simulink model "sysgenQAMExt"  (Simulink 7.7)
settings: Solver=ode45  StartTime=0.0  StopTime=3000  RelTol=1e-3
PreLoadFcn:
  | xlrequire('PreLoadFcn')
values from neighbouring files (symbols this model uses):
  hh = hh1/max(hh1)    [sysgenCostasLoop_PreLoadFcn.m]
  j = find(xLabel==')')    [sdspfscope2_r13.m]
  k = (k-1)*3+2    [sdspfscope2_r13.m]
  mu = xfix({xlSigned, 18, 15, xlRound, xlSaturate}, mu)    [lmsErr.m]
undefined symbols (not defined in the file or in its folder): chan, k_i0, k_p0, xlipgetpartsetting, xlsfunxy
libraries: xbsIndex_r4 x477, simulink x2, dspsigops x2, dspmlti4 x2, commchan3 x1, xbsCopyrightNotice_r4 x1, dspobslib x1
(part 2 of 5)

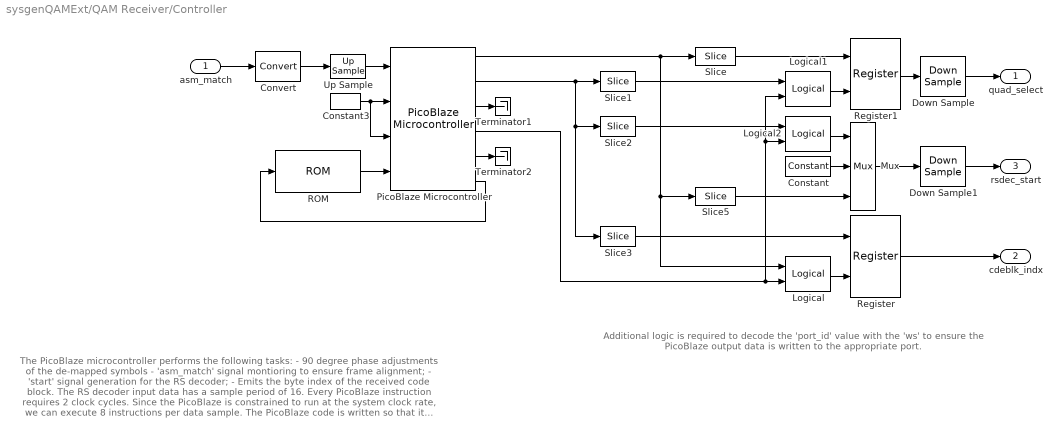
== system sysgenQAMExt/QAM Receiver/Controller ==
  note: The PicoBlaze microcontroller performs the following tasks:
      |
      | - 90 degree phase adjustments of the de-mapped symbols
      | - 'asm_match' signal montioring to ensure frame alignment;
      | - 'start' signal generation for the RS decoder;
      | - Emits the byte index of the received code block.
      |
      | The RS decoder input data has a sample period of 16.
      | Every PicoBlaze instruction requires 2 clock cycles.  Since
      | the PicoBlaze is constrained to run at the system clock rate,
      | we can execute 8 instructions per data sample.  The
      | PicoBlaze code is  written so that it remains synchronized
      | with the data, i.e. there are exactly eight instructions between
      | input samples.
      |
      | Please refer to the PicoBlaze code, sysgenQAMExt.psm for
      | more information.
  note: Additional logic is required to decode the
      | 'port_id' value with the 'ws' to ensure
      | the PicoBlaze output data is written
      | to the appropriate port.
  asm_match : Inport
  Constant : xbsIndex_r4/Constant  const=0  gui_display_data_type=Fixed-point  arith_type=Boolean  n_bits=1  bin_pt=0  preci_type=Single  exp_width=8  frac_width=24  explicit_period=off  period=1  equ=P=C  opselect=C  inp2=PCIN>>17  opr=+  inp1=P  carry=CIN  dbl_ovrd=off  block_type=constant
      settings: block_version=VER_STRING_GOES_HERE
  Constant3 : xbsIndex_r4/Constant  const=0  gui_display_data_type=Fixed-point  arith_type=Boolean  n_bits=1  bin_pt=0  preci_type=Single  exp_width=8  frac_width=24  explicit_period=on  period=1  equ=P=C  opselect=C  inp2=PCIN>>17  opr=+  inp1=P  carry=CIN  dbl_ovrd=off  block_type=constant
      settings: block_version=VER_STRING_GOES_HERE
  Convert : xbsIndex_r4/Convert  gui_display_data_type=Fixed-point  arith_type=Unsigned  n_bits=8  bin_pt=0  float_type=Single  exp_bits=8  fraction_bits=24  quantization=Truncate  overflow=Wrap  en=off  latency=0  dbl_ovrd=off  pipeline=off  block_type=convert
      settings: infoedit=The input is presented at the output after quantization and overflow effects.<P><P>Hardware notes: Additional hardware is used when rounding or saturation is selected and output width is less than the input width.  xl_area=[0, 0, 0, 0, 0, 0, 0]  block_version=VER_STRING_GOES_HERE
  Down Sample : xbsIndex_r4/Down Sample  sample_ratio=4  sample_phase="Last Value of Frame  (most efficient)"  en=off  latency=1  dbl_ovrd=off  block_type=dsamp
      settings: xl_area=[0, 0, 0, 0, 0, 0, 0]  block_version=VER_STRING_GOES_HERE
  Down Sample1 : xbsIndex_r4/Down Sample  sample_ratio=16  sample_phase="Last Value of Frame  (most efficient)"  en=off  latency=1  dbl_ovrd=off  block_type=dsamp
      settings: xl_area=[0, 0, 0, 0, 0, 0, 0]  block_version=VER_STRING_GOES_HERE
  Logical : xbsIndex_r4/Logical  logical_function=AND  inputs=2  en=off  latency=0  precision=Full  arith_type=Unsigned  n_bits=8  bin_pt=2  align_bp=on  dbl_ovrd=off  block_type=logical
      settings: xl_area=[0, 0, 0, 0, 0, 0, 0]  block_version=VER_STRING_GOES_HERE
  Logical1 : xbsIndex_r4/Logical  logical_function=AND  inputs=2  en=off  latency=0  precision=Full  arith_type=Unsigned  n_bits=8  bin_pt=2  align_bp=on  dbl_ovrd=off  block_type=logical
      settings: xl_area=[0, 0, 0, 0, 0, 0, 0]  block_version=VER_STRING_GOES_HERE
  Logical2 : xbsIndex_r4/Logical  logical_function=AND  inputs=2  en=off  latency=0  precision=Full  arith_type=Unsigned  n_bits=8  bin_pt=2  align_bp=on  dbl_ovrd=off  block_type=logical
      settings: xl_area=[0, 0, 0, 0, 0, 0, 0]  block_version=VER_STRING_GOES_HERE
  Mux : xbsIndex_r4/Mux  inputs=2  en=off  latency=0  precision=Full  arith_type="Signed  (2's comp)"  n_bits=8  bin_pt=2  quantization=Truncate  overflow=Wrap  dbl_ovrd=off  block_type=mux
      settings: xl_area=[0, 0, 0, 0, 0, 0, 0]  block_version=VER_STRING_GOES_HERE
  PicoBlaze Microcontroller : xbsIndex_r4/PicoBlaze Microcontroller  version=PicoBlaze 3  display_mi=off  xl_view_as=Decimal  block_type=pb
      settings: xl_area=[0, 0, 0, 0, 0, 0, 0]  block_version=VER_STRING_GOES_HERE
  ROM : xbsIndex_r4/ROM  depth=2^10  initVector=sysgenQAMExt_PBInstructs  distributed_mem=Block RAM  rst=off  init_reg=0  en=off  latency=1  gui_display_data_type=Fixed-point  arith_type=Unsigned  n_bits=18  bin_pt=0  preci_type=Single  exp_width=8  frac_width=24  dbl_ovrd=off  optimize=Area  use_rpm=off  block_type=sprom
      settings: xl_area=[0, 0, 0, 0, 0, 0, 0]  block_version=VER_STRING_GOES_HERE
  Register : xbsIndex_r4/Register  init=0  rst=off  en=on  dbl_ovrd=off  block_type=register
      settings: xl_area=[0, 0, 0, 0, 0, 0, 0]  block_version=VER_STRING_GOES_HERE
  Register1 : xbsIndex_r4/Register  init=0  rst=off  en=on  dbl_ovrd=off  block_type=register
      settings: xl_area=[0, 0, 0, 0, 0, 0, 0]  block_version=VER_STRING_GOES_HERE
  Slice : xbsIndex_r4/Slice  nbits=2  boolean_output=off  mode=Lower Bit Location + Width  bit1=0  base1=MSB of Input  bit0=0  base0=LSB of Input  dbl_ovrd=off  block_type=slice
      settings: infoedit="Extracts a given range of bits from each input sample and presents it at the output.  The output type is ordinarily unsigned with binary point at zero, but can be Boolean when the slice is one bit wide.<P><P>Hardware notes: In hardware this block costs nothing."  block_version=VER_STRING_GOES_HERE
  Slice1 : xbsIndex_r4/Slice  nbits=1  boolean_output=on  mode=Lower Bit Location + Width  bit1=0  base1=MSB of Input  bit0=0  base0=LSB of Input  dbl_ovrd=off  block_type=slice
      settings: infoedit="Extracts a given range of bits from each input sample and presents it at the output.  The output type is ordinarily unsigned with binary point at zero, but can be Boolean when the slice is one bit wide.<P><P>Hardware notes: In hardware this block costs nothing."  block_version=VER_STRING_GOES_HERE
  Slice2 : xbsIndex_r4/Slice  nbits=1  boolean_output=on  mode=Lower Bit Location + Width  bit1=0  base1=MSB of Input  bit0=1  base0=LSB of Input  dbl_ovrd=off  block_type=slice
      settings: infoedit="Extracts a given range of bits from each input sample and presents it at the output.  The output type is ordinarily unsigned with binary point at zero, but can be Boolean when the slice is one bit wide.<P><P>Hardware notes: In hardware this block costs nothing."  block_version=VER_STRING_GOES_HERE
  Slice3 : xbsIndex_r4/Slice  nbits=1  boolean_output=on  mode=Lower Bit Location + Width  bit1=0  base1=MSB of Input  bit0=2  base0=LSB of Input  dbl_ovrd=off  block_type=slice
      settings: infoedit="Extracts a given range of bits from each input sample and presents it at the output.  The output type is ordinarily unsigned with binary point at zero, but can be Boolean when the slice is one bit wide.<P><P>Hardware notes: In hardware this block costs nothing."  block_version=VER_STRING_GOES_HERE
  Slice5 : xbsIndex_r4/Slice  nbits=1  boolean_output=on  mode=Lower Bit Location + Width  bit1=0  base1=MSB of Input  bit0=0  base0=LSB of Input  dbl_ovrd=off  block_type=slice
      settings: infoedit="Extracts a given range of bits from each input sample and presents it at the output.  The output type is ordinarily unsigned with binary point at zero, but can be Boolean when the slice is one bit wide.<P><P>Hardware notes: In hardware this block costs nothing."  block_version=VER_STRING_GOES_HERE
  Terminator1 : Terminator
  Terminator2 : Terminator
  Up Sample : xbsIndex_r4/Up Sample  sample_ratio=16  copy_samples=on  en=off  latency=0  dbl_ovrd=off  block_type=usamp
      settings: infoedit="Up samples input data.  Inserted values  can be zeros or copies of the most recent input sample.<P><P>Hardware notes: No hardware is needed if inserted values are copies of the input sample; otherwise, a mux and single bit flip-flop are used."  xl_area=[0, 0, 0, 0, 0, 0, 0]  block_version=VER_STRING_GOES_HERE
  quad_select : Outport
  cdeblk_indx : Outport  Port=2
  rsdec_start : Outport  Port=3
  wires:
  PicoBlaze Microcontroller/3 -> Terminator1/1
  PicoBlaze Microcontroller/2 -> Slice1/1, Slice2/1, Slice3/1
  ROM/1 -> PicoBlaze Microcontroller/4
  Down Sample/1 -> quad_select/1
  Down Sample1/1 -> rsdec_start/1
  Register/1 -> cdeblk_indx/1
  PicoBlaze Microcontroller/1 -> Slice/1, Register/1, Slice5/1
  Slice3/1 -> Logical/1
  PicoBlaze Microcontroller/4 -> Logical/2, Logical1/2, Logical2/2
  Logical/1 -> Register/2
  Slice1/1 -> Logical1/1
  Logical2/1 -> Mux/1
  Slice2/1 -> Logical2/1
  Constant/1 -> Mux/2
  Slice5/1 -> Mux/3
  Mux/1 -> Down Sample1/1
  Slice/1 -> Register1/1
  Logical1/1 -> Register1/2
  Register1/1 -> Down Sample/1
  asm_match/1 -> Convert/1
  Up Sample/1 -> PicoBlaze Microcontroller/1
  Convert/1 -> Up Sample/1
  PicoBlaze Microcontroller/6 -> ROM/1
  PicoBlaze Microcontroller/5 -> Terminator2/1
  Constant3/1 -> PicoBlaze Microcontroller/2, PicoBlaze Microcontroller/3

== system sysgenQAMExt/QAM Receiver/Frame Aligner ==
  note: Register block 'Offset Capture' captures the current value
      | of the 'Offset Counter' block when the ASM is detected.
      | This captured value is used to drive the 'addr' ports of the
      | 'align match' and 'align dout' addressable shift register (ASR)
      | blocks.  By adjusting the ASR address values, the serial data
      | is shifted appropriately so that it aligns correctly to the byte
      | boundaries in the serial to parallel converter.
      |
      | The data is aligned so that the first received bit of the ASM
      | becomes the MSB of the corresponding byte output.
  note: The 'ASM Matcher' subsystem asserts an
      | 'asm_match' output signal when the ASM
      | bit pattern is succesfully matched.  The
      | 'dout' port presents a delayed (32 cycles)
      | version  'din' signal.
  din : Inport
  ASM Matcher : Subsystem
  Convert : xbsIndex_r4/Convert  gui_display_data_type=Fixed-point  arith_type=Unsigned  n_bits=1  bin_pt=0  float_type=Single  exp_bits=8  fraction_bits=24  quantization=Truncate  overflow=Wrap  en=off  latency=0  dbl_ovrd=off  pipeline=off  block_type=convert
      settings: infoedit=The input is presented at the output after quantization and overflow effects.<P><P>Hardware notes: Additional hardware is used when rounding or saturation is selected and output width is less than the input width.  xl_area=[0, 0, 0, 0, 0, 0, 0]  block_version=VER_STRING_GOES_HERE
  Delay1 : xbsIndex_r4/Delay  rst=off  infoeditControl=Selection of Reset will increase slice count due to use of real FFs and instead of SRLs  en=off  latency=32  dbl_ovrd=off  reg_retiming=off  block_type=delay
      settings: infoedit="Delay line having  configurable length.<P><P>Hardware notes: A delay line is a chain, each link of which is an SRL16 followed by a flip-flop. If register retiming is enabled, the delay line is a chain of flip-flops."  xl_area=[0, 0, 0, 0, 0, 0, 0]  block_version=VER_STRING_GOES_HERE
  Down Sample : xbsIndex_r4/Down Sample  sample_ratio=8  sample_phase="Last Value of Frame  (most efficient)"  en=off  latency=1  dbl_ovrd=off  block_type=dsamp
      settings: xl_area=[0, 0, 0, 0, 0, 0, 0]  block_version=VER_STRING_GOES_HERE
  Offset Counter : xbsIndex_r4/Counter  cnt_type=Free Running  cnt_to=Inf  operation=Down  start_count=6  cnt_by_val=1  arith_type=Unsigned  n_bits=3  bin_pt=0  load_pin=off  rst=off  en=off  explicit_period=off  period=2  dbl_ovrd=off  use_behavioral_HDL=off  implementation=Fabric  use_rpm=off  block_type=counter
      settings: infoedit="Configurable up, down and up/down counter.<P><P>Hardware notes: Free running counters are the least expensive in hardware.  A count limited counter is implemented by combining a counter with a comparator."  xl_area=[0, 0, 0, 0, 0, 0, 0]  block_version=VER_STRING_GOES_HERE
  Offset Capture : xbsIndex_r4/Register  init=0  rst=off  en=on  dbl_ovrd=off  block_type=register
      settings: xl_area=[0, 0, 0, 0, 0, 0, 0]  block_version=VER_STRING_GOES_HERE
  Serial to Parallel : xbsIndex_r4/Serial to Parallel  input_order=Most Significant Word First  arith_type=Unsigned  output_bits=8  bin_pt=0  rst=off  en=off  latency=1  dbl_ovrd=off  block_type=s2p
      settings: infoedit=Groups of samples presented serially at the input become single samples presented at the output.  xl_area=[0, 0, 0, 0, 0, 0, 0]  block_version=VER_STRING_GOES_HERE
  align dout : xbsIndex_r4/Addressable Shift Register  infer_latency=on  depth=2  initVector=[0]  en=off  dbl_ovrd=off  use_behavioral_HDL=off  Optimization=Resource  use_rpm=off  block_type=addrsr
      settings: infoedit="Delay of configurable length.  Any element in the delay line can be addressed and driven onto the output port.<P><P>Hardware notes: Implemented using SRL16s.  If a Virtex-II device is used, multiple SRLC16s are cascaded together."  xl_area=[0, 0, 0, 0, 0, 0, 0]  block_version=VER_STRING_GOES_HERE
  align match : xbsIndex_r4/Addressable Shift Register  infer_latency=on  depth=2  initVector=[0]  en=off  dbl_ovrd=off  use_behavioral_HDL=off  Optimization=Resource  use_rpm=off  block_type=addrsr
      settings: infoedit="Delay of configurable length.  Any element in the delay line can be addressed and driven onto the output port.<P><P>Hardware notes: Implemented using SRL16s.  If a Virtex-II device is used, multiple SRLC16s are cascaded together."  xl_area=[0, 0, 0, 0, 0, 0, 0]  block_version=VER_STRING_GOES_HERE
  dout : Outport
  match : Outport  Port=2
  wires:
  align dout/1 -> Serial to Parallel/1
  Serial to Parallel/1 -> dout/1
  din/1 -> ASM Matcher/1(din)
  Offset Counter/1 -> Offset Capture/1
  ASM Matcher/1(asm_match) -> Offset Capture/2, Delay1/1
  Delay1/1 -> align match/1
  align match/1 -> Down Sample/1
  Down Sample/1 -> Convert/1
  Convert/1 -> match/1
  ASM Matcher/2(dout) -> align dout/1
  Offset Capture/1 -> align match/2, align dout/2

== system sysgenQAMExt/QAM Receiver/QAM Demodulator ==
  x_i : Inport
  x_q : Inport  Port=2
  quad_select : Inport  Port=3
  Adaptive Equalizer : Subsystem
  Carrier Recovery : Subsystem
  Error : Scope
      settings: TimeRange=500  YMin=-35  YMax=-7.5
  Rotate and De-map : Subsystem
  Terminator : Terminator
  Terminator1 : Terminator
  dB : Subsystem
  demap_I : Outport
  demap_Q : Outport  Port=2
  wires:
  Adaptive Equalizer/2(dhat_I) -> Carrier Recovery/1(dhat_I)
  Adaptive Equalizer/3(dhat_Q) -> Carrier Recovery/2(dhat_Q)
  Carrier Recovery/1(sym_I) -> Adaptive Equalizer/3(sym_I)
  Carrier Recovery/2(sym_Q) -> Adaptive Equalizer/4(sym_Q)
  Adaptive Equalizer/1(err_n) -> dB/1(In)
  x_i/1 -> Adaptive Equalizer/1(x_i)
  x_q/1 -> Adaptive Equalizer/2(x_q)
  dB/1(Out) -> Error/1
  Adaptive Equalizer/4(coef) -> Terminator/1
  Carrier Recovery/3(constellation) -> Terminator1/1
  Carrier Recovery/4(qntzd_I) -> Rotate and De-map/1(qntzd_I)
  Carrier Recovery/5(qntzd_Q) -> Rotate and De-map/2(qntzd_Q)
  quad_select/1 -> Rotate and De-map/3(quad_sel)
  Rotate and De-map/1(demap_I) -> demap_I/1
  Rotate and De-map/2(demap_Q) -> demap_Q/1

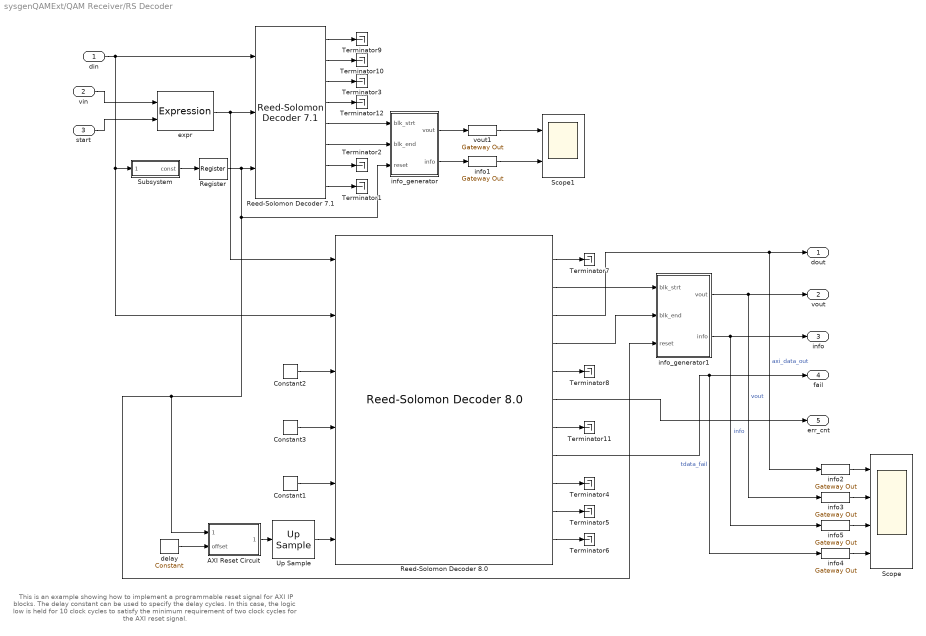
== system sysgenQAMExt/QAM Receiver/RS Decoder ==
  note: This is an example showing how to implement a programmable reset signal
      |  for AXI IP blocks. The delay constant can be used to specify the delay cycles.
      | In this case, the logic low is held for 10 clock cycles to satisfy the minimum
      | requirement of two clock cycles for the AXI reset signal.
  din : Inport
  vin : Inport  Port=2
  start : Inport  Port=3
  AXI Reset Circuit : Subsystem
  Constant1 : xbsIndex_r4/Constant  const=1  gui_display_data_type=Boolean  arith_type=Boolean  n_bits=16  bin_pt=14  preci_type=Single  exp_width=8  frac_width=24  explicit_period=on  period=16  equ=P=C  opselect=C  inp2=PCIN>>17  opr=+  inp1=P  carry=CIN  dbl_ovrd=off  block_type=constant
      settings: block_version=12.3
  Constant2 : xbsIndex_r4/Constant  const=0  gui_display_data_type=Boolean  arith_type=Boolean  n_bits=16  bin_pt=14  preci_type=Single  exp_width=8  frac_width=24  explicit_period=on  period=16  equ=P=C  opselect=C  inp2=PCIN>>17  opr=+  inp1=P  carry=CIN  dbl_ovrd=off  block_type=constant
      settings: block_version=12.3
  Constant3 : xbsIndex_r4/Constant  const=1  gui_display_data_type=Boolean  arith_type=Boolean  n_bits=16  bin_pt=14  preci_type=Single  exp_width=8  frac_width=24  explicit_period=on  period=16  equ=P=C  opselect=C  inp2=PCIN>>17  opr=+  inp1=P  carry=CIN  dbl_ovrd=off  block_type=constant
      settings: block_version=12.3
  "Reed-Solomon Decoder 7.1 " : xbsIndex_r4/Reed-Solomon Decoder 7.1   code_specification=CCSDS  symbol_width=8  field_polynomial=391  scaling_factor=11  generator_start=112  variable_block_length=off  symbols_per_block=255  data_symbols=239  variable_number_of_check_symbols=off  define_supported_r_in_values=off  number_of_supported_r_in_values=2  supported_r_in_definition_file='no_coe_file_loaded'  optimization=Speed  self_recovering=off  memory_style=Automatic  clocks_per_symbol=1  number_of_channels=1  number_of_puncture_patterns=0  puncture_definition_file='no_coe_file_loaded'  clock_enable=off  info_end=off  synchronous_reset=on  original_delayed_data=off  erase=off  error_statistics=off  marker_bits=off  number_of_marker_bits=1  ip_name=Reed-Solomon Decoder  ip_version=7.1  dsptool_ready=false  ipcore_usecache=true  ipcore_useipmodelcache=true  wrapper_available=true  port_translation_map={ 'ce' => 'en', 'sr' => 'rst'}  structural_sim=true  ipcore_do_not_force_period=true  block_type=rs_decoder_v7_1
  "Reed-Solomon Decoder 8.0 " : xbsIndex_r4/Reed-Solomon Decoder 8.0   code_specification=CCSDS  symbol_width=8  field_polynomial=391  scaling_factor=11  generator_start=112  variable_block_length=off  symbols_per_block=255  data_symbols=239  variable_number_of_check_symbols=off  define_supported_r_in_values=off  number_of_supported_r_in_values=2  supported_r_in_definition_file='no_coe_file_loaded'  self_recovering=off  memory_style=Automatic  number_of_channels=1  output_check_symbols=on  number_of_puncture_patterns=0  puncture_definition_file='no_coe_file_loaded'  aclken=off  info=off  aresetn=on  original_delayed_data=off  erase=off  error_statistics=off  marker_bits=off  number_of_marker_bits=1  trim_axipin_name=off  ip_name=Reed-Solomon Decoder  ip_version=8.0  dsptool_ready=false  ipcore_usecache=true  ipcore_useipmodelcache=true  wrapper_available=true  port_translation_map={ 'aclken' => 'en', 'aresetn' => 'rst'}  structural_sim=true  ipcore_do_not_force_period=true  block_type=rs_decoder_v8_0
  Register : xbsIndex_r4/Register  init=1  rst=off  en=off  dbl_ovrd=off  block_type=register
      settings: block_version=VER_STRING_GOES_HERE
  Scope : Scope  NumInputPorts=4
      settings: YMin=-5~-5~-5~-5  YMax=5~5~5~5  SaveName=ScopeData2
  Scope1 : Scope  NumInputPorts=2
      settings: YMin=-5~-5  YMax=5~5  SaveName=ScopeData3
  Subsystem : Subsystem
  Terminator{1..12} (12 alike) : Terminator
  Up Sample : xbsIndex_r4/Up Sample  sample_ratio=16  copy_samples=on  en=off  latency=0  dbl_ovrd=off  block_type=usamp
  delay : xbsIndex_r4/Constant  const=10  gui_display_data_type=Fixed-point  arith_type=Unsigned  n_bits=8  bin_pt=0  preci_type=Single  exp_width=8  frac_width=24  explicit_period=on  period=16  equ=P=C  opselect=C  inp2=PCIN>>17  opr=+  inp1=P  carry=CIN  dbl_ovrd=off  block_type=constant
      settings: block_version=9.2.01
  expr : xbsIndex_r4/Expression  expression=a & b  align_bp=on  en=off  latency=0  precision=Full  arith_type=Unsigned  n_bits=8  bin_pt=2  dbl_ovrd=off  block_type=expr
      settings: block_version=VER_STRING_GOES_HERE
  info{1..5} (5 alike) : xbsIndex_r4/Gateway Out  inherit_from_input=off  hdl_port=off  timing_constraint=None  locs_specified=off  LOCs={}  UseAsDAC=off  DACChannel='1'  block_type=gatewayout
      settings: infoedit="Gateway out block.  Converts Xilinx fixed point or floating-point type inputs into ouputs of type Simulink integer, double, or fixed point.<br><br>Hardware notes:  In hardware these blocks become top level output ports or are discarded, depending on how they are configured."
  info_generator : Subsystem  mask{sym_width=8, kk=239}
      mask prompts: sym_width "Symbol Width"; kk "Number of information symbols per code block"
      settings: CopyFcn=set_param(gcb, 'LinkStatus', 'none');
  info_generator1 : Subsystem  mask{sym_width=8, kk=239}
      mask prompts: sym_width "Symbol Width"; kk "Number of information symbols per code block"
      settings: CopyFcn=set_param(gcb, 'LinkStatus', 'none');
  vout1 : xbsIndex_r4/Gateway Out  inherit_from_input=off  hdl_port=off  timing_constraint=None  locs_specified=off  LOCs={}  UseAsDAC=off  DACChannel='1'  block_type=gatewayout
      settings: infoedit="Gateway out block.  Converts Xilinx fixed point or floating-point type inputs into ouputs of type Simulink integer, double, or fixed point.<br><br>Hardware notes:  In hardware these blocks become top level output ports or are discarded, depending on how they are configured."
  dout : Outport
  vout : Outport  Port=2
  info : Outport  Port=3
  fail : Outport  Port=4
  err_cnt : Outport  Port=5
  wires:
  info_generator/1(vout) -> vout1/1
  info_generator/2(info) -> info1/1
  start/1 -> expr/2
  vin/1 -> expr/1
  expr/1 -> "Reed-Solomon Decoder 7.1 "/2, "Reed-Solomon Decoder 8.0 "/1
  Subsystem/1(const) -> Register/1
  din/1 -> "Reed-Solomon Decoder 7.1 "/1, Subsystem/1(sample), "Reed-Solomon Decoder 8.0 "/2
  "Reed-Solomon Decoder 7.1 "/7 -> Terminator2/1
  "Reed-Solomon Decoder 7.1 "/8 -> Terminator1/1
  "Reed-Solomon Decoder 7.1 "/6 -> info_generator/2(blk_end)
  "Reed-Solomon Decoder 7.1 "/3 -> Terminator3/1
  "Reed-Solomon Decoder 7.1 "/5 -> info_generator/1(blk_strt)
  Register/1 -> "Reed-Solomon Decoder 7.1 "/3, info_generator/3(reset), info_generator1/3(reset), AXI Reset Circuit/1(valid_in)
  Constant1/1 -> "Reed-Solomon Decoder 8.0 "/5
  Constant2/1 -> "Reed-Solomon Decoder 8.0 "/3
  "Reed-Solomon Decoder 8.0 "/2 -> info_generator1/1(blk_strt)
  "Reed-Solomon Decoder 8.0 "/4 -> info_generator1/2(blk_end)
  "Reed-Solomon Decoder 8.0 "/6 -> err_cnt/1
  "Reed-Solomon Decoder 8.0 "/11 -> Terminator6/1
  "Reed-Solomon Decoder 8.0 "/10 -> Terminator5/1
  "Reed-Solomon Decoder 8.0 "/9 -> Terminator4/1
  "Reed-Solomon Decoder 8.0 "/5 -> Terminator8/1
  "Reed-Solomon Decoder 8.0 "/1 -> Terminator7/1
  Constant3/1 -> "Reed-Solomon Decoder 8.0 "/4
  "Reed-Solomon Decoder 8.0 "/3 -> dout/1, info2/1  "axi_data_out"
  "Reed-Solomon Decoder 8.0 "/8 -> fail/1, info4/1  "tdata_fail"
  info_generator1/1(vout) -> vout/1, info3/1  "vout"
  info_generator1/2(info) -> info/1, info5/1  "info"
  info1/1 -> Scope1/2
  vout1/1 -> Scope1/1
  "Reed-Solomon Decoder 7.1 "/1 -> Terminator9/1
  "Reed-Solomon Decoder 7.1 "/2 -> Terminator10/1
  "Reed-Solomon Decoder 8.0 "/7 -> Terminator11/1
  info2/1 -> Scope/1
  info3/1 -> Scope/2
  info5/1 -> Scope/3
  info4/1 -> Scope/4
  delay/1 -> AXI Reset Circuit/2(offset)
  "Reed-Solomon Decoder 7.1 "/4 -> Terminator12/1
  AXI Reset Circuit/1(valid_out) -> Up Sample/1
  Up Sample/1 -> "Reed-Solomon Decoder 8.0 "/6

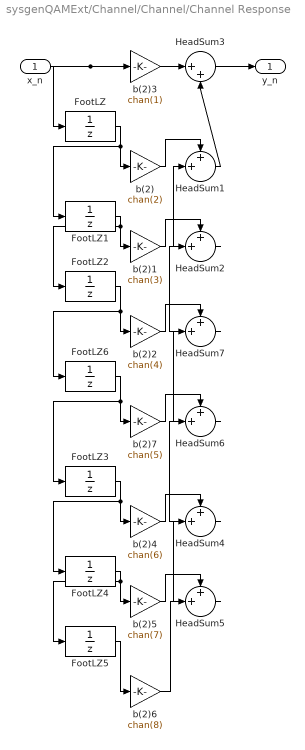
== system sysgenQAMExt/Channel/Channel/Channel Response ==
  x_n : Inport
  FootLZ : UnitDelay
  FootLZ{1..2,4..6} (5 alike) : UnitDelay  SampleTime=-1
  FootLZ3 : UnitDelay
  HeadSum{1..2,4..7} (6 alike) : Sum  Inputs=++|  SaturateOnIntegerOverflow=on  InputSameDT=on  OutDataTypeStr=Inherit: Same as first input
  HeadSum3 : Sum  Inputs=|++  SaturateOnIntegerOverflow=on  InputSameDT=on  OutDataTypeStr=Inherit: Same as first input
  b(2) : Gain  Gain=chan(2)  SaturateOnIntegerOverflow=on  OutDataTypeStr=Inherit: Same as input  ParamDataTypeStr=Inherit: Same as input
  b(2)1 : Gain  Gain=chan(3)  SaturateOnIntegerOverflow=on  OutDataTypeStr=Inherit: Same as input  ParamDataTypeStr=Inherit: Same as input
  b(2)2 : Gain  Gain=chan(4)  SaturateOnIntegerOverflow=on  OutDataTypeStr=Inherit: Same as input  ParamDataTypeStr=Inherit: Same as input
  b(2)3 : Gain  Gain=chan(1)  SaturateOnIntegerOverflow=on  OutDataTypeStr=Inherit: Same as input  ParamDataTypeStr=Inherit: Same as input
  b(2)4 : Gain  Gain=chan(6)  SaturateOnIntegerOverflow=on  OutDataTypeStr=Inherit: Same as input  ParamDataTypeStr=Inherit: Same as input
  b(2)5 : Gain  Gain=chan(7)  SaturateOnIntegerOverflow=on  OutDataTypeStr=Inherit: Same as input  ParamDataTypeStr=Inherit: Same as input
  b(2)6 : Gain  Gain=chan(8)  SaturateOnIntegerOverflow=on  OutDataTypeStr=Inherit: Same as input  ParamDataTypeStr=Inherit: Same as input
  b(2)7 : Gain  Gain=chan(5)  SaturateOnIntegerOverflow=on  OutDataTypeStr=Inherit: Same as input  ParamDataTypeStr=Inherit: Same as input
  y_n : Outport
  wires:
  HeadSum3/1 -> y_n/1
  HeadSum1/1 -> HeadSum3/2
  b(2)3/1 -> HeadSum3/1
  x_n/1 -> b(2)3/1, FootLZ/1
  HeadSum2/1 -> HeadSum1/2
  b(2)1/1 -> HeadSum2/1
  b(2)/1 -> HeadSum1/1
  FootLZ1/1 -> b(2)1/1, FootLZ2/1
  FootLZ/1 -> FootLZ1/1, b(2)/1
  FootLZ2/1 -> b(2)2/1, FootLZ6/1
  b(2)7/1 -> HeadSum6/1
  b(2)6/1 -> HeadSum5/2
  HeadSum5/1 -> HeadSum4/2
  b(2)5/1 -> HeadSum5/1
  b(2)4/1 -> HeadSum4/1
  FootLZ5/1 -> b(2)6/1
  FootLZ4/1 -> b(2)5/1, FootLZ5/1
  FootLZ3/1 -> FootLZ4/1, b(2)4/1
  FootLZ6/1 -> b(2)7/1, FootLZ3/1
  b(2)2/1 -> HeadSum7/1
  HeadSum7/1 -> HeadSum2/2
  HeadSum4/1 -> HeadSum6/2
  HeadSum6/1 -> HeadSum7/2

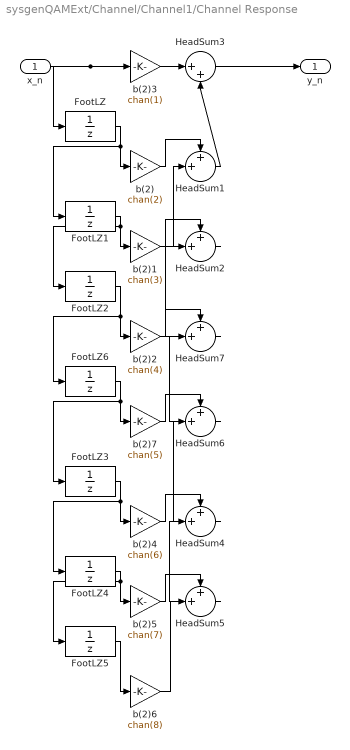
== system sysgenQAMExt/Channel/Channel1/Channel Response ==
  x_n : Inport
  FootLZ : UnitDelay
  FootLZ{1..2,4..6} (5 alike) : UnitDelay  SampleTime=-1
  FootLZ3 : UnitDelay
  HeadSum{1..2,4..7} (6 alike) : Sum  Inputs=++|  SaturateOnIntegerOverflow=on  InputSameDT=on  OutDataTypeStr=Inherit: Same as first input
  HeadSum3 : Sum  Inputs=|++  SaturateOnIntegerOverflow=on  InputSameDT=on  OutDataTypeStr=Inherit: Same as first input
  b(2) : Gain  Gain=chan(2)  SaturateOnIntegerOverflow=on  OutDataTypeStr=Inherit: Same as input  ParamDataTypeStr=Inherit: Same as input
  b(2)1 : Gain  Gain=chan(3)  SaturateOnIntegerOverflow=on  OutDataTypeStr=Inherit: Same as input  ParamDataTypeStr=Inherit: Same as input
  b(2)2 : Gain  Gain=chan(4)  SaturateOnIntegerOverflow=on  OutDataTypeStr=Inherit: Same as input  ParamDataTypeStr=Inherit: Same as input
  b(2)3 : Gain  Gain=chan(1)  SaturateOnIntegerOverflow=on  OutDataTypeStr=Inherit: Same as input  ParamDataTypeStr=Inherit: Same as input
  b(2)4 : Gain  Gain=chan(6)  SaturateOnIntegerOverflow=on  OutDataTypeStr=Inherit: Same as input  ParamDataTypeStr=Inherit: Same as input
  b(2)5 : Gain  Gain=chan(7)  SaturateOnIntegerOverflow=on  OutDataTypeStr=Inherit: Same as input  ParamDataTypeStr=Inherit: Same as input
  b(2)6 : Gain  Gain=chan(8)  SaturateOnIntegerOverflow=on  OutDataTypeStr=Inherit: Same as input  ParamDataTypeStr=Inherit: Same as input
  b(2)7 : Gain  Gain=chan(5)  SaturateOnIntegerOverflow=on  OutDataTypeStr=Inherit: Same as input  ParamDataTypeStr=Inherit: Same as input
  y_n : Outport
  wires:
  HeadSum3/1 -> y_n/1
  HeadSum1/1 -> HeadSum3/2
  b(2)3/1 -> HeadSum3/1
  x_n/1 -> b(2)3/1, FootLZ/1
  HeadSum2/1 -> HeadSum1/2
  b(2)1/1 -> HeadSum2/1
  b(2)/1 -> HeadSum1/1
  FootLZ1/1 -> b(2)1/1, FootLZ2/1
  FootLZ/1 -> FootLZ1/1, b(2)/1
  HeadSum4/1 -> HeadSum6/2
  b(2)7/1 -> HeadSum6/1
  b(2)6/1 -> HeadSum5/2
  HeadSum5/1 -> HeadSum4/2
  b(2)5/1 -> HeadSum5/1
  b(2)4/1 -> HeadSum4/1
  FootLZ5/1 -> b(2)6/1
  FootLZ4/1 -> b(2)5/1, FootLZ5/1
  FootLZ3/1 -> FootLZ4/1, b(2)4/1
  FootLZ2/1 -> b(2)2/1, FootLZ6/1
  FootLZ6/1 -> FootLZ3/1, b(2)7/1
  HeadSum6/1 -> HeadSum7/2
  HeadSum7/1 -> HeadSum2/2
  b(2)2/1 -> HeadSum7/1

== system sysgenQAMExt/FEC and QAM Symbol Mapping/RS Encoder/Subsystem1 ==
  ufix_vout : Inport
  ufix_rfd : Inport  Port=2
  sel : Inport  Port=3
  Constant1 : xbsIndex_r4/Constant  const=0  gui_display_data_type=Fixed-point  arith_type=Boolean  n_bits=1  bin_pt=0  preci_type=Single  exp_width=8  frac_width=24  explicit_period=off  period=1  equ=P=C  opselect=C  inp2=PCIN>>17  opr=+  inp1=P  carry=CIN  dbl_ovrd=off  block_type=constant
      settings: block_version=VER_STRING_GOES_HERE
  Constant2 : xbsIndex_r4/Constant  const=1  gui_display_data_type=Fixed-point  arith_type=Boolean  n_bits=1  bin_pt=0  preci_type=Single  exp_width=8  frac_width=24  explicit_period=off  period=1  equ=P=C  opselect=C  inp2=PCIN>>17  opr=+  inp1=P  carry=CIN  dbl_ovrd=off  block_type=constant
      settings: block_version=VER_STRING_GOES_HERE
  Convert : xbsIndex_r4/Convert  gui_display_data_type=Fixed-point  arith_type=Boolean  n_bits=1  bin_pt=0  float_type=Single  exp_bits=8  fraction_bits=24  quantization=Truncate  overflow=Wrap  en=off  latency=0  dbl_ovrd=off  pipeline=off  block_type=convert
      settings: infoedit=The input is presented at the output after quantization and overflow effects.<P><P>Hardware notes: Additional hardware is used when rounding or saturation is selected and output width is less than the input width.  block_version=VER_STRING_GOES_HERE
  Convert1 : xbsIndex_r4/Convert  gui_display_data_type=Fixed-point  arith_type=Boolean  n_bits=1  bin_pt=0  float_type=Single  exp_bits=8  fraction_bits=24  quantization=Truncate  overflow=Wrap  en=off  latency=0  dbl_ovrd=off  pipeline=off  block_type=convert
      settings: infoedit=The input is presented at the output after quantization and overflow effects.<P><P>Hardware notes: Additional hardware is used when rounding or saturation is selected and output width is less than the input width.  block_version=VER_STRING_GOES_HERE
  Mux : xbsIndex_r4/Mux  inputs=2  en=off  latency=0  precision=Full  arith_type=Unsigned  n_bits=8  bin_pt=2  quantization=Truncate  overflow=Wrap  dbl_ovrd=off  block_type=mux
      settings: block_version=VER_STRING_GOES_HERE
  Mux1 : xbsIndex_r4/Mux  inputs=2  en=off  latency=0  precision=Full  arith_type=Unsigned  n_bits=8  bin_pt=2  quantization=Truncate  overflow=Wrap  dbl_ovrd=off  block_type=mux
      settings: block_version=VER_STRING_GOES_HERE
  bool_vout : Outport
  bool_rfd : Outport  Port=2
  wires:
  Mux/1 -> Convert/1
  Mux1/1 -> Convert1/1
  Constant1/1 -> Mux/2
  Constant2/1 -> Mux1/2
  sel/1 -> Mux1/1, Mux/1
  Convert/1 -> bool_vout/1
  ufix_vout/1 -> Mux/3
  Convert1/1 -> bool_rfd/1
  ufix_rfd/1 -> Mux1/3

== system sysgenQAMExt/FEC and QAM Symbol Mapping/RS Encoder/Subsystem2 ==
  sample : Inport
  Constant3 : xbsIndex_r4/Constant  const=1  gui_display_data_type=Fixed-point  arith_type=Unsigned  n_bits=1  bin_pt=0  preci_type=Single  exp_width=8  frac_width=24  explicit_period=off  period=1  equ=P=C  opselect=C  inp2=PCIN>>17  opr=+  inp1=P  carry=CIN  dbl_ovrd=off  block_type=constant
      settings: dsp48_infoedit="The use of this block for DSP48 instructions is deprecated.  Please use the Opcode block."  block_version=VER_STRING_GOES_HERE
  Convert2 : xbsIndex_r4/Convert  gui_display_data_type=Fixed-point  arith_type=Unsigned  n_bits=1  bin_pt=0  float_type=Single  exp_bits=8  fraction_bits=24  quantization=Truncate  overflow=Wrap  en=off  latency=0  dbl_ovrd=off  pipeline=off  block_type=convert
      settings: infoedit=The input is presented at the output after quantization and overflow effects.<P><P>Hardware notes: Additional hardware is used when rounding or saturation is selected and output width is less than the input width.  block_version=VER_STRING_GOES_HERE
  expr1 : xbsIndex_r4/Expression  expression=a | b  align_bp=on  en=off  latency=0  precision=Full  arith_type=Unsigned  n_bits=8  bin_pt=2  dbl_ovrd=off  block_type=expr
      settings: block_version=VER_STRING_GOES_HERE
  const : Outport
  wires:
  Constant3/1 -> expr1/2
  Convert2/1 -> expr1/1
  sample/1 -> Convert2/1
  expr1/1 -> const/1

== system sysgenQAMExt/QAM Receiver/Frame Aligner/ASM Matcher ==
  note: The 32-bit ASM pattern is matched using parallel comparators.
      | The subsystem includes 4 subsystems that match a byte at a time.
  din : Inport
  Concat : xbsIndex_r4/Concat  num_inputs=2  dbl_ovrd=off  block_type=concat
      settings: block_version=VER_STRING_GOES_HERE
  Concat1 : xbsIndex_r4/Concat  num_inputs=2  dbl_ovrd=off  block_type=concat
      settings: block_version=VER_STRING_GOES_HERE
  Concat2 : xbsIndex_r4/Concat  num_inputs=2  dbl_ovrd=off  block_type=concat
      settings: block_version=VER_STRING_GOES_HERE
  Convert : xbsIndex_r4/Convert  gui_display_data_type=Fixed-point  arith_type=Boolean  n_bits=8  bin_pt=6  float_type=Single  exp_bits=8  fraction_bits=24  quantization=Truncate  overflow=Wrap  en=off  latency=0  dbl_ovrd=off  pipeline=off  block_type=convert
      settings: infoedit=The input is presented at the output after quantization and overflow effects.<P><P>Hardware notes: Additional hardware is used when rounding or saturation is selected and output width is less than the input width.  xl_area=[0, 0, 0, 0, 0, 0, 0]  block_version=VER_STRING_GOES_HERE
  Delay2 : xbsIndex_r4/Delay  rst=off  infoeditControl=Selection of Reset will increase slice count due to use of real FFs and instead of SRLs  en=off  latency=1  dbl_ovrd=off  reg_retiming=off  block_type=delay
      settings: infoedit="Delay line having  configurable length.<P><P>Hardware notes: A delay line is a chain, each link of which is an SRL16 followed by a flip-flop. If register retiming is enabled, the delay line is a chain of flip-flops."  xl_area=[0, 0, 0, 0, 0, 0, 0]  block_version=VER_STRING_GOES_HERE
  ROM : xbsIndex_r4/ROM  depth=16  initVector=[zeros(1,15) 1]  distributed_mem=Distributed memory  rst=off  init_reg=0  en=off  latency=0  gui_display_data_type=Fixed-point  arith_type=Unsigned  n_bits=1  bin_pt=0  preci_type=Single  exp_width=8  frac_width=24  dbl_ovrd=off  optimize=Area  use_rpm=off  block_type=sprom
      settings: xl_area=[0, 0, 0, 0, 0, 0, 0]  block_version=VER_STRING_GOES_HERE
  asm_comp4 : Subsystem  mask{byte_comp=26}
      mask prompts: byte_comp "Byte"
  asm_comp_1 : Subsystem  mask{byte_comp=29}
      mask prompts: byte_comp "Byte"
  asm_comp_2 : Subsystem  mask{byte_comp=252}
      mask prompts: byte_comp "Byte"
  asm_comp_3 : Subsystem  mask{byte_comp=207}
      mask prompts: byte_comp "Byte"
  asm_match : Outport
  dout : Outport  Port=2
  wires:
  din/1 -> asm_comp_1/1(din)
  asm_comp_1/1(dout) -> asm_comp_2/1(din)
  asm_comp_2/1(dout) -> asm_comp_3/1(din)
  asm_comp_3/1(dout) -> asm_comp4/1(din)
  asm_comp4/1(dout) -> Delay2/1
  asm_comp_1/2(match) -> Concat/1
  asm_comp_2/2(match) -> Concat/2
  Concat/1 -> Concat1/1
  asm_comp_3/2(match) -> Concat1/2
  Concat1/1 -> Concat2/1
  asm_comp4/2(match) -> Concat2/2
  ROM/1 -> Convert/1
  Concat2/1 -> ROM/1
  Convert/1 -> asm_match/1
  Delay2/1 -> dout/1

== system sysgenQAMExt/QAM Receiver/QAM Demodulator/Adaptive Equalizer ==
  note: Adaptive equalizers operate in a receiver to minimize intersymbol interference (ISI), due to
      | channel-induced distortion, of the received signal. The equalizer operates in cascade with
      | a matched filter (MF), synchronous sampler, and decision device (slicer) operating at the
      | symbol rate. A gradient descent process such as the least-mean square (LMS) algorithm
      | adjusts the equalizer weights to minimize the difference between the input and output of
      | the decision device.
      |
      | In the case of an adaptive decision directed (DD) channel equalizer the desired signal is
      | produced by utilizing the known structure of the system alphabet.  A 8-tap decision directed
      | equalizer using an LMS coefficient update is used in this model. The input samples are
      | complex valued quantities as are the filter weights and the output signal.
      |
      | A fractionally spaced equalizer (FSE) sampling at a rate of two samples per symbol is
      | used to avoid aliasing.  The equalizer is a multirate structure that is most efficiently
      | implemented using a polyphase decimator architecture.  For this model, two
      | polyphase arms are used.
      |
      | Additional information on adaptive equalizers and FSE can be found at:
      |
      | Haykin, S. "Adaptive Filter Theory"  Prentice Hall, New Jersey, 1996.
      |
      | J.R. Treichler, I. Fijalkow, and C.R. Johnson, Jr.  "Fractionally Spaced
      | Equalizers"  IEEE Signal Processing Magazine, May 1996, pp. 65-81.
  note: The LMS Error Calc subsystem determines
      | the error between the filter approximation of
      | the received symbol and the hard decision.
      | The real and imaginary error is weighted
      | against the adaptation rate constant, and fed
      | back to the equalizer ALU.
  note: Note the absence of the slicer in the equalizer.  The Doppler content
      | of the filter output signal prevents a slicer from being used to drive the
      | decision directed LMS coefficient update.  The decisions used in the
      | LMS Error Calc subsystem must be available at the same rotation rate,
      | and direction, as the received constellation.   The decisions are
      | therefore generated in the Carrier Recovery subsystem and are fed
      | back to the equalizer.
  x_i : Inport
  x_q : Inport  Port=2
  sym_I : Inport  Port=3
  sym_Q : Inport  Port=4
  ALU : Subsystem
  CNVRT3 : xbsIndex_r4/Convert  gui_display_data_type=Fixed-point  arith_type="Signed  (2's comp)"  n_bits=18  bin_pt=14  float_type=Single  exp_bits=8  fraction_bits=24  quantization="Round  (unbiased: +/- Inf)"  overflow=Wrap  en=off  latency=0  dbl_ovrd=off  pipeline=off  block_type=convert
      settings: infoedit=The input is presented at the output after quantization and overflow effects.<P><P>Hardware notes: Additional hardware is used when rounding or saturation is selected and output width is less than the input width.  xl_area=[0, 0, 0, 0, 0, 0, 0]  block_version=VER_STRING_GOES_HERE
  CNVRT4 : xbsIndex_r4/Convert  gui_display_data_type=Fixed-point  arith_type="Signed  (2's comp)"  n_bits=18  bin_pt=14  float_type=Single  exp_bits=8  fraction_bits=24  quantization="Round  (unbiased: +/- Inf)"  overflow=Wrap  en=off  latency=0  dbl_ovrd=off  pipeline=off  block_type=convert
      settings: infoedit=The input is presented at the output after quantization and overflow effects.<P><P>Hardware notes: Additional hardware is used when rounding or saturation is selected and output width is less than the input width.  xl_area=[0, 0, 0, 0, 0, 0, 0]  block_version=VER_STRING_GOES_HERE
  Delay{1..4} (4 alike) : xbsIndex_r4/Delay  rst=off  infoeditControl=Selection of Reset will increase slice count due to use of real FFs and instead of SRLs  en=off  latency=1  dbl_ovrd=off  reg_retiming=off  block_type=delay
      settings: infoedit="Delay line having  configurable length.<P><P>Hardware notes: A delay line is a chain, each link of which is an SRL16 followed by a flip-flop. If register retiming is enabled, the delay line is a chain of flip-flops."  xl_area=[0, 0, 0, 0, 0, 0, 0]  block_version=VER_STRING_GOES_HERE
  Delay8 : xbsIndex_r4/Delay  rst=off  infoeditControl=Selection of Reset will increase slice count due to use of real FFs and instead of SRLs  en=off  latency=k-7  dbl_ovrd=off  reg_retiming=off  block_type=delay
      settings: infoedit="Delay line having  configurable length.<P><P>Hardware notes: A delay line is a chain, each link of which is an SRL16 followed by a flip-flop. If register retiming is enabled, the delay line is a chain of flip-flops."  xl_area=[0, 0, 0, 0, 0, 0, 0]  block_version=VER_STRING_GOES_HERE
  Delay9 : xbsIndex_r4/Delay  rst=off  infoeditControl=Selection of Reset will increase slice count due to use of real FFs and instead of SRLs  en=off  latency=k-7  dbl_ovrd=off  reg_retiming=off  block_type=delay
      settings: infoedit="Delay line having  configurable length.<P><P>Hardware notes: A delay line is a chain, each link of which is an SRL16 followed by a flip-flop. If register retiming is enabled, the delay line is a chain of flip-flops."  xl_area=[0, 0, 0, 0, 0, 0, 0]  block_version=VER_STRING_GOES_HERE
  LMS Error Calc : Subsystem
  err_n : Outport
  dhat_I : Outport  Port=2
  dhat_Q : Outport  Port=3
  coef : Outport  Port=4
  wires:
  ALU/2(dhat_Q) -> Delay9/1
  x_i/1 -> Delay4/1
  x_q/1 -> Delay2/1
  Delay4/1 -> Delay1/1
  Delay2/1 -> Delay3/1
  Delay1/1 -> ALU/1(x_I)
  Delay3/1 -> ALU/2(x_Q)
  LMS Error Calc/3(err_n) -> err_n/1
  Delay9/1 -> CNVRT4/1, LMS Error Calc/2(dhat_Q)
  sym_I/1 -> LMS Error Calc/3(det_I)
  sym_Q/1 -> LMS Error Calc/4(det_Q)
  LMS Error Calc/1(muErr_I) -> ALU/3(err_I)
  LMS Error Calc/2(muErr_Q) -> ALU/4(err_Q)
  ALU/1(dhat_I) -> Delay8/1
  Delay8/1 -> LMS Error Calc/1(dhat_I), CNVRT3/1
  CNVRT3/1 -> dhat_I/1
  CNVRT4/1 -> dhat_Q/1
  ALU/3(Coeff) -> coef/1

== system sysgenQAMExt/QAM Receiver/QAM Demodulator/Carrier Recovery ==
  note: Every complex multiplier in the model is
      | implemented using 4 dedicated Virtex-II
      | multipliers and 2 adders.
  note: The Doppler content of the signal means that the equalizer slicer cannot be used
      | to drive the decision directed LMS coefficient update.  The required decisions must
      | be supplied by the detector in the carrier recovery loop.  Further, these decisions
      | must be available at the same rotation rate, and direction, as the received constellation.
      | To achieve this, the DDS output is conjugated to produce a heterodyning signal
      | that up-converts the CRL hard decisions. This waveform is supplied to the equalizer
      | LMS processor.
  note: The Phase Detector subsystem strips the modulation
      | from the received signal and produces a signal proportional
      | to the phase difference between the locally generated
      | quadrature carriers and those of the received signal.
  note: The DPLL employs a proportional plus integral
      | loop filter formed by a scaled digital integrator
      | and a scaled direct path.
  dhat_I : Inport
  dhat_Q : Inport  Port=2
  Cmplx Mult : Subsystem
  Cmplx Mult1 : Subsystem
  Constant : xbsIndex_r4/Constant  const=1  gui_display_data_type=Fixed-point  arith_type=Boolean  n_bits=1  bin_pt=0  preci_type=Single  exp_width=8  frac_width=24  explicit_period=off  period=1  equ=P=C  opselect=C  inp2=PCIN>>17  opr=+  inp1=P  carry=CIN  dbl_ovrd=off  block_type=constant
      settings: block_version=VER_STRING_GOES_HERE
  DDS : Subsystem
  DPLL Loop Filter : Subsystem
  Gateway Out1 : xbsIndex_r4/Gateway Out  inherit_from_input=off  hdl_port=off  timing_constraint="Data Rate;  Set 'FAST' Attribute"  locs_specified=off  LOCs={}  UseAsDAC=off  DACChannel='1'  block_type=gatewayout
      settings: infoedit="Gateway out block.  Converts Xilinx fixed point inputs into ouputs of type Simulink integer, double, or fixed point.<P><P>Hardware notes:  In hardware these blocks become top level output ports or are discarded, depending on how they are configured."  xl_area=[0, 0, 0, 0, 0, 0, 0]  block_version=VER_STRING_GOES_HERE
  Gateway Out2 : xbsIndex_r4/Gateway Out  inherit_from_input=off  hdl_port=off  timing_constraint="Data Rate;  Set 'FAST' Attribute"  locs_specified=off  LOCs={}  UseAsDAC=off  DACChannel='1'  block_type=gatewayout
      settings: infoedit="Gateway out block.  Converts Xilinx fixed point inputs into ouputs of type Simulink integer, double, or fixed point.<P><P>Hardware notes:  In hardware these blocks become top level output ports or are discarded, depending on how they are configured."  xl_area=[0, 0, 0, 0, 0, 0, 0]  block_version=VER_STRING_GOES_HERE
  Negate : xbsIndex_r4/Negate  precision=Full  arith_type=Unsigned  n_bits=8  bin_pt=2  quantization=Truncate  overflow=Wrap  en=off  latency=0  dbl_ovrd=off  block_type=negate
      settings: xl_area=[0, 0, 0, 0, 0, 0, 0]  block_version=VER_STRING_GOES_HERE
  Phase Detector : Subsystem
  Real-Imag to Complex2 : RealImagToComplex
  sym_I : Outport
  sym_Q : Outport  Port=2
  constellation : Outport  Port=3
  qntzd_I : Outport  Port=4
  qntzd_Q : Outport  Port=5
  wires:
  Cmplx Mult/1(p_r) -> Gateway Out1/1, Phase Detector/1(I_in)
  dhat_Q/1 -> Cmplx Mult/2(a_i)
  dhat_I/1 -> Cmplx Mult/1(a_r)
  Cmplx Mult/2(p_i) -> Gateway Out2/1, Phase Detector/2(Q_in)
  Gateway Out1/1 -> Real-Imag to Complex2/1
  Gateway Out2/1 -> Real-Imag to Complex2/2
  Real-Imag to Complex2/1 -> constellation/1
  Cmplx Mult1/2(p_i) -> sym_Q/1
  Phase Detector/3(phs_err) -> DPLL Loop Filter/1(phs_err)
  Phase Detector/1(det_I) -> Cmplx Mult1/1(a_r)
  Phase Detector/2(det_Q) -> Cmplx Mult1/2(a_i)
  Cmplx Mult1/1(p_r) -> sym_I/1
  DDS/2(Out2) -> Cmplx Mult/3(b_r), Cmplx Mult1/3(b_r)
  DDS/1(Out1) -> Negate/1, Cmplx Mult1/4(b_i)
  DPLL Loop Filter/1(y) -> DDS/1(In1)
  Constant/1 -> DDS/2(In2)
  Negate/1 -> Cmplx Mult/4(b_i)
  Phase Detector/4(qntzd_I) -> qntzd_I/1
  Phase Detector/5(qntzd_Q) -> qntzd_Q/1

== system sysgenQAMExt/QAM Receiver/QAM Demodulator/Rotate and De-map ==
  note: This subsystem performs de-mapping on the 16-QAM symbols.  The 'quad_sel' signal
      | determines whether the hard decisions are rotated 0, 90, 180, or 270 degrees before
      | they are de-mapped.
  qntzd_I : Inport
  qntzd_Q : Inport  Port=2
  quad_sel : Inport  Port=3
  Mux : xbsIndex_r4/Mux  inputs=4  en=off  latency=1  precision=Full  arith_type="Signed  (2's comp)"  n_bits=8  bin_pt=2  quantization=Truncate  overflow=Wrap  dbl_ovrd=off  block_type=mux
      settings: xl_area=[0, 0, 0, 0, 0, 0, 0]  block_version=VER_STRING_GOES_HERE
  Mux1 : xbsIndex_r4/Mux  inputs=4  en=off  latency=1  precision=Full  arith_type="Signed  (2's comp)"  n_bits=8  bin_pt=2  quantization=Truncate  overflow=Wrap  dbl_ovrd=off  block_type=mux
      settings: xl_area=[0, 0, 0, 0, 0, 0, 0]  block_version=VER_STRING_GOES_HERE
  Negate : xbsIndex_r4/Negate  precision=User Defined  arith_type="Signed  (2's comp)"  n_bits=3  bin_pt=1  quantization=Truncate  overflow=Wrap  en=off  latency=0  dbl_ovrd=off  block_type=negate
      settings: xl_area=[0, 0, 0, 0, 0, 0, 0]  block_version=VER_STRING_GOES_HERE
  Negate1 : xbsIndex_r4/Negate  precision=User Defined  arith_type="Signed  (2's comp)"  n_bits=3  bin_pt=1  quantization=Truncate  overflow=Wrap  en=off  latency=0  dbl_ovrd=off  block_type=negate
      settings: xl_area=[0, 0, 0, 0, 0, 0, 0]  block_version=VER_STRING_GOES_HERE
  ROM : xbsIndex_r4/ROM  depth=8  initVector=[0 0 1 0 0 0 3 2]  distributed_mem=Block RAM  rst=off  init_reg=0  en=off  latency=1  gui_display_data_type=Fixed-point  arith_type=Unsigned  n_bits=2  bin_pt=0  preci_type=Single  exp_width=8  frac_width=24  dbl_ovrd=off  optimize=Area  use_rpm=off  block_type=sprom
      settings: xl_area=[0, 0, 0, 0, 0, 0, 0]  block_version=VER_STRING_GOES_HERE
  ROM1 : xbsIndex_r4/ROM  depth=8  initVector=[0 0 1 0 0 0 3 2]  distributed_mem=Block RAM  rst=off  init_reg=0  en=off  latency=1  gui_display_data_type=Fixed-point  arith_type=Unsigned  n_bits=2  bin_pt=0  preci_type=Single  exp_width=8  frac_width=24  dbl_ovrd=off  optimize=Area  use_rpm=off  block_type=sprom
      settings: xl_area=[0, 0, 0, 0, 0, 0, 0]  block_version=VER_STRING_GOES_HERE
  Reinterpret1 : xbsIndex_r4/Reinterpret  force_arith_type=on  arith_type=Unsigned  force_bin_pt=on  bin_pt=0  block_type=cast
      settings: infoedit="Changes type of samples without altering their binary representation.<P><P>Hardware notes: In hardware this block costs nothing.<P><P>Example:  Suppose the input is 6 bits wide, signed, with 2 fractional bits, and the output is forced to unsigned with 0 fractional bits.  Then an input of -2.0 (1110.00 in binary 2's complement) becomes an output of 56 (111000 in binary)."  block_version=VER_STRING_GOES_HERE
  Reinterpret2 : xbsIndex_r4/Reinterpret  force_arith_type=on  arith_type=Unsigned  force_bin_pt=on  bin_pt=0  block_type=cast
      settings: infoedit="Changes type of samples without altering their binary representation.<P><P>Hardware notes: In hardware this block costs nothing.<P><P>Example:  Suppose the input is 6 bits wide, signed, with 2 fractional bits, and the output is forced to unsigned with 0 fractional bits.  Then an input of -2.0 (1110.00 in binary 2's complement) becomes an output of 56 (111000 in binary)."  block_version=VER_STRING_GOES_HERE
  demap_I : Outport
  demap_Q : Outport  Port=2
  wires:
  ROM1/1 -> demap_Q/1
  quad_sel/1 -> Mux/1, Mux1/1
  qntzd_I/1 -> Negate/1, Mux/2, Mux1/5
  qntzd_Q/1 -> Mux1/2, Mux/3, Negate1/1
  Negate/1 -> Mux/4, Mux1/3
  Mux/1 -> Reinterpret2/1
  Mux1/1 -> Reinterpret1/1
  ROM/1 -> demap_I/1
  Reinterpret1/1 -> ROM1/1
  Reinterpret2/1 -> ROM/1
  Negate1/1 -> Mux/5, Mux1/4

== system sysgenQAMExt/QAM Receiver/QAM Demodulator/dB ==
  In : Inport
  Abs : Abs  SaturateOnIntegerOverflow=on
  Constant : Constant  Value=0
  Constant1 : Constant
  Constant2 : Constant
  Gain1 : Gain  Gain=20  SaturateOnIntegerOverflow=on  OutDataTypeStr=Inherit: Same as input  ParamDataTypeStr=Inherit: Same as input
  Multiport Switch : MultiPortSwitch  Inputs=2  zeroidx=off  SaturateOnIntegerOverflow=on  InputSameDT=on
  Relational Operator : RelationalOperator  Operator===  InputSameDT=on
  Sum : Sum  Inputs=|++  SaturateOnIntegerOverflow=on  InputSameDT=on  OutDataTypeStr=Inherit: Same as first input
  log10 : Math  Operator=log10  SaturateOnIntegerOverflow=on
  Out : Outport
  wires:
  Multiport Switch/1 -> log10/1
  Constant1/1 -> Multiport Switch/3
  Constant/1 -> Relational Operator/1
  Abs/1 -> Multiport Switch/2, Relational Operator/2
  Constant2/1 -> Sum/2
  Sum/1 -> Multiport Switch/1
  Relational Operator/1 -> Sum/1
  Gain1/1 -> Out/1
  In/1 -> Abs/1
  log10/1 -> Gain1/1
